simulink model "ALL_JP360_DBW_V6_5_1103"  (R2022a)
settings: Solver=FixedStepAuto  StartTime=0.0  StopTime=inf  FixedStep=0.01  RelTol=1e-3  EnableMultiTasking=on
model workspace (MAT data in the model file):
  g = 9.8
undefined symbols (not defined in the file or in its folder): canChannel, delta_v_p, IPM_Line_C0, IPM_Line_C1, IPM_Line_C2, IPM_Line_C3, M, M_p, MRR_ObjDistX, MRR_ObjDistY, MRR_ObjFusionCamID, MRR_ObjFusionSig, MRR_ObjID, MRR_ObjRelVelX, MRR_ObjRelVelY, MRR_ObjType, MRR_ObjUpdFlg, none, obj_vaild, untracktime, V, videoinput
libraries: canfdmsglib x230, canfdlib x76, slpidlib x24, simulink x18, dspstat3 x14, ctrlSharedLib x1, simulink_extras x1, imaqlib x1, realtime_pacer_lib x1, dspvision x1, visionsinks x1
(part 10 of 55)

== system ALL_JP360_DBW_V6_5_1103/MsgFromCAN/CCAN_ADCU_MsgFromCAN/CCAN_ADCU_ESP_Pressure_0x241 ==
  CCAN_ADCU_ESP_Pressure_0x241FromInData : Inport  OutDataTypeStr=Bus:CAN_FD_MESSAGE_BUS
  Bus Creator : BusCreator  Inputs=11  OutDataTypeStr=Bus:CCAN_ADCU_ESP_Pressure_0x241  NonVirtualBus=on
  CAN FD Unpack : canfdmsglib/CAN FD Unpack  CANdbFile=HiFire_JPT360_CCAN_Matrix_CAN_V1.72_VP_ADCU.dbc  MsgList=(none)  MsgName=ESP_Pressure_0x241  ProtocolMode=CAN FD  MsgIDType=Standard (11-bit identifier)  MsgIdentifier=577  MsgLength=8  SignalInfo={'ABS_ForbidRegen_Active','54','1','BE','unsigned','Standard','0','1','0','0','1';'Checksum_0x241','56','8','BE','unsigned','Standard','0','1','0','0','255';'ESP_Master_Cylinder_Pressure','12','12','BE','unsigned','Standard','0','0.0625','0','0','255.9375';'ESP_Master_Cylinder_Pressure_Status','55','1','BE','unsigned','Standard','0','1','0','0','1';'ESP_MbRegenTargetWhl','32','16','BE','unsigned','Standard','0','1','-30000','-30000','30000';'ESP_MbRegenTargetWhlQualifier','52','2','BE','unsigned','Standard','0','1','0','0','2';'ESP_PresOffsetMasterCylinder','43','5','BE','unsigned','Standard','0','1','-15','-15','15';'ESP_PresOffsetMasterCylinderValid','42','1','BE','unsigned','Standard','0','1','0','0','1';'ESP_TrfCaseModReqdByEsp','40','2','BE','unsigned','Standard','0','1','0','0','3';'ESP_TrfCaseTqLmtdByEsp','16','12','BE','unsigned','Standard','0','1','0','0','4095';'RollingCounter_0x241','48','4','BE','unsigned','Standard','0','1','0','0','15'}  IDPort=off  TimestampPort=off  ErrorPort=off  RemotePort=off  LengthPort=off  StatusPort=off  BRSPort=off  ESIPort=off  DLCPort=off  ApplyMinMax=off
      settings: SourceProductBaseCode=XP,ME,VN  DataFormat=CANdb specified signals
  Data Type Conversion1 : DataTypeConversion  OutDataTypeStr=boolean  SaturateOnIntegerOverflow=off  RndMeth=Floor
  Data Type Conversion10 : DataTypeConversion  OutDataTypeStr=int16  SaturateOnIntegerOverflow=off  RndMeth=Floor
  Data Type Conversion{6..7,9,11} (4 alike) : DataTypeConversion  OutDataTypeStr=int8  SaturateOnIntegerOverflow=off  RndMeth=Floor
  Data Type Conversion2 : DataTypeConversion  OutDataTypeStr=uint8  SaturateOnIntegerOverflow=off  RndMeth=Floor
  Data Type Conversion3 : DataTypeConversion  OutDataTypeStr=single  SaturateOnIntegerOverflow=off  RndMeth=Floor
  Data Type Conversion4 : DataTypeConversion  OutDataTypeStr=boolean  SaturateOnIntegerOverflow=off  RndMeth=Floor
  Data Type Conversion5 : DataTypeConversion  OutDataTypeStr=int16  SaturateOnIntegerOverflow=off  RndMeth=Floor
  Data Type Conversion8 : DataTypeConversion  OutDataTypeStr=boolean  SaturateOnIntegerOverflow=off  RndMeth=Floor
  CCAN_ADCU_ESP_Pressure_0x241FromOutData : Outport  OutDataTypeStr=Bus:CCAN_ADCU_ESP_Pressure_0x241
  wires:
  CAN FD Unpack/1 -> Data Type Conversion1/1
  CAN FD Unpack/2 -> Data Type Conversion2/1
  CAN FD Unpack/3 -> Data Type Conversion3/1
  CAN FD Unpack/4 -> Data Type Conversion4/1
  CAN FD Unpack/5 -> Data Type Conversion5/1
  CAN FD Unpack/6 -> Data Type Conversion6/1
  CAN FD Unpack/7 -> Data Type Conversion7/1
  CAN FD Unpack/8 -> Data Type Conversion8/1
  CAN FD Unpack/9 -> Data Type Conversion9/1
  CAN FD Unpack/10 -> Data Type Conversion10/1
  CAN FD Unpack/11 -> Data Type Conversion11/1
  Data Type Conversion1/1 -> Bus Creator/1  "ABS_ForbidRegen_Active"
  Data Type Conversion2/1 -> Bus Creator/2  "Checksum_0x241"
  Data Type Conversion3/1 -> Bus Creator/3  "ESP_Master_Cylinder_Pressure"
  Data Type Conversion4/1 -> Bus Creator/4  "ESP_Master_Cylinder_Pressure_Status"
  Data Type Conversion5/1 -> Bus Creator/5  "ESP_MbRegenTargetWhl"
  Data Type Conversion6/1 -> Bus Creator/6  "ESP_MbRegenTargetWhlQualifier"
  Data Type Conversion7/1 -> Bus Creator/7  "ESP_PresOffsetMasterCylinder"
  Data Type Conversion8/1 -> Bus Creator/8  "ESP_PresOffsetMasterCylinderValid"
  Data Type Conversion9/1 -> Bus Creator/9  "ESP_TrfCaseModReqdByEsp"
  Data Type Conversion10/1 -> Bus Creator/10  "ESP_TrfCaseTqLmtdByEsp"
  Data Type Conversion11/1 -> Bus Creator/11  "RollingCounter_0x241"
  Bus Creator/1 -> CCAN_ADCU_ESP_Pressure_0x241FromOutData/1  "CCAN_ADCU_ESP_Pressure_0x241FromOutData"
  CCAN_ADCU_ESP_Pressure_0x241FromInData/1 -> CAN FD Unpack/1  "CCAN_ADCU_ESP_Pressure_0x241FromInData"

== system ALL_JP360_DBW_V6_5_1103/MsgFromCAN/CCAN_ADCU_MsgFromCAN/CCAN_ADCU_ESP_RAW_0x212 ==
  CCAN_ADCU_ESP_RAW_0x212FromInData : Inport  OutDataTypeStr=Bus:CAN_FD_MESSAGE_BUS
  Bus Creator : BusCreator  Inputs=10  OutDataTypeStr=Bus:CCAN_ADCU_ESP_RAW_0x212  NonVirtualBus=on
  CAN FD Unpack : canfdmsglib/CAN FD Unpack  CANdbFile=HiFire_JPT360_CCAN_Matrix_CAN_V1.72_VP_ADCU.dbc  MsgList=(none)  MsgName=ESP_RAW_0x212  ProtocolMode=CAN FD  MsgIDType=Standard (11-bit identifier)  MsgIdentifier=530  MsgLength=8  SignalInfo={'Checksum_0x212','56','8','BE','unsigned','Standard','0','1','0','0','255';'ESP_vxwWheelFLValid','55','1','BE','unsigned','Standard','0','1','0','0','1';'ESP_vxwWheelFRValid','54','1','BE','unsigned','Standard','0','1','0','0','1';'ESP_vxwWheelRLValid','53','1','BE','unsigned','Standard','0','1','0','0','1';'ESP_vxwWheelRRValid','52','1','BE','unsigned','Standard','0','1','0','0','1';'ESP_vxwWheelRawFL','12','12','BE','unsigned','Standard','0','0.05625','0','0','230.2875';'ESP_vxwWheelRawFR','16','12','BE','unsigned','Standard','0','0.05625','0','0','230.2875';'ESP_vxwWheelRawRL','36','12','BE','unsigned','Standard','0','0.05625','0','0','230.2875';'ESP_vxwWheelRawRR','40','12','BE','unsigned','Standard','0','0.05625','0','0','230.2875';'RollingCounter_0x212','48','4','BE','unsigned','Standard','0','1','0','0','15'}  IDPort=off  TimestampPort=off  ErrorPort=off  RemotePort=off  LengthPort=off  StatusPort=off  BRSPort=off  ESIPort=off  DLCPort=off  ApplyMinMax=off
      settings: SourceProductBaseCode=XP,ME,VN  DataFormat=CANdb specified signals
  Data Type Conversion1 : DataTypeConversion  OutDataTypeStr=uint8  SaturateOnIntegerOverflow=off  RndMeth=Floor
  Data Type Conversion10 : DataTypeConversion  OutDataTypeStr=int8  SaturateOnIntegerOverflow=off  RndMeth=Floor
  Data Type Conversion{2..5} (4 alike) : DataTypeConversion  OutDataTypeStr=boolean  SaturateOnIntegerOverflow=off  RndMeth=Floor
  Data Type Conversion{6..9} (4 alike) : DataTypeConversion  OutDataTypeStr=single  SaturateOnIntegerOverflow=off  RndMeth=Floor
  CCAN_ADCU_ESP_RAW_0x212FromOutData : Outport  OutDataTypeStr=Bus:CCAN_ADCU_ESP_RAW_0x212
  wires:
  CAN FD Unpack/1 -> Data Type Conversion1/1
  CAN FD Unpack/2 -> Data Type Conversion2/1
  CAN FD Unpack/3 -> Data Type Conversion3/1
  CAN FD Unpack/4 -> Data Type Conversion4/1
  CAN FD Unpack/5 -> Data Type Conversion5/1
  CAN FD Unpack/6 -> Data Type Conversion6/1
  CAN FD Unpack/7 -> Data Type Conversion7/1
  CAN FD Unpack/8 -> Data Type Conversion8/1
  CAN FD Unpack/9 -> Data Type Conversion9/1
  CAN FD Unpack/10 -> Data Type Conversion10/1
  Data Type Conversion1/1 -> Bus Creator/1  "Checksum_0x212"
  Data Type Conversion2/1 -> Bus Creator/2  "ESP_vxwWheelFLValid"
  Data Type Conversion3/1 -> Bus Creator/3  "ESP_vxwWheelFRValid"
  Data Type Conversion4/1 -> Bus Creator/4  "ESP_vxwWheelRLValid"
  Data Type Conversion5/1 -> Bus Creator/5  "ESP_vxwWheelRRValid"
  Data Type Conversion6/1 -> Bus Creator/6  "ESP_vxwWheelRawFL"
  Data Type Conversion7/1 -> Bus Creator/7  "ESP_vxwWheelRawFR"
  Data Type Conversion8/1 -> Bus Creator/8  "ESP_vxwWheelRawRL"
  Data Type Conversion9/1 -> Bus Creator/9  "ESP_vxwWheelRawRR"
  Data Type Conversion10/1 -> Bus Creator/10  "RollingCounter_0x212"
  Bus Creator/1 -> CCAN_ADCU_ESP_RAW_0x212FromOutData/1  "CCAN_ADCU_ESP_RAW_0x212FromOutData"
  CCAN_ADCU_ESP_RAW_0x212FromInData/1 -> CAN FD Unpack/1  "CCAN_ADCU_ESP_RAW_0x212FromInData"

== system ALL_JP360_DBW_V6_5_1103/MsgFromCAN/CCAN_ADCU_MsgFromCAN/CCAN_ADCU_ESP_Status_0x243 ==
  CCAN_ADCU_ESP_Status_0x243FromInData : Inport  OutDataTypeStr=Bus:CAN_FD_MESSAGE_BUS
  Bus Creator : BusCreator  Inputs=38  OutDataTypeStr=Bus:CCAN_ADCU_ESP_Status_0x243  NonVirtualBus=on
  CAN FD Unpack : canfdmsglib/CAN FD Unpack  CANdbFile=HiFire_JPT360_CCAN_Matrix_CAN_V1.72_VP_ADCU.dbc  MsgList=(none)  MsgName=ESP_Status_0x243  ProtocolMode=CAN FD  MsgIDType=Standard (11-bit identifier)  MsgIdentifier=579  MsgLength=8  SignalInfo={'ABS_HAZActive','2','1','BE','unsigned','Standard','0','1','0','0','1';'Checksum_0x243','56','8','BE','unsigned','Standard','0','1','0','0','255';'EBS_EbsFlgFlt','43','1','BE','unsigned','Standard','0','1','0','0','1';'ESP_ATS_Driving_mode_confirm','28','4','BE','unsigned','Standard','0','1','0','0','15';'ESP_ATS_Fault_mode','27','1','BE','unsigned','Standard','0','1','0','0','1';'ESP_ATS_failure_Lamp','24','3','BE','unsigned','Standard','0','1','0','0','7';'ESP_AVHWarningMessage','20','1','BE','unsigned','Standard','0','1','0','0','1';'ESP_AvhActive','21','1','BE','unsigned','Standard','0','1','0','0','1';'ESP_AvhAvabliable','23','1','BE','unsigned','Standard','0','1','0','0','1';'ESP_AvhStandby','22','1','BE','unsigned','Standard','0','1','0','0','1';'ESP_CCSwitchOff','8','1','BE','unsigned','Standard','0','1','0','0','1';'ESP_CdpActive','15','1','BE','unsigned','Standard','0','1','0','0','1';'ESP_CdpAvailable','14','1','BE','unsigned','Standard','0','1','0','0','1';'ESP_Driving_mode_req','36','4','BE','unsigned','Standard','0','1','0','0','15';'ESP_EPBErrorStatus','6','2','BE','unsigned','Standard','0','1','0','0','3';'ESP_EPBStatus','3','3','BE','unsigned','Standard','0','1','0','0','7';'ESP_EPBWarningMessage1','19','1','BE','unsigned','Standard','0','1','0','0','1';'ESP_EPBWarningMessage2','18','1','BE','unsigned','Standard','0','1','0','0','1';'ESP_EPBWarningMessage3','17','1','BE','unsigned','Standard','0','1','0','0','1';'ESP_ESPInfoLamp','44','1','BE','unsigned','Standard','0','1','0','0','1';'ESP_EspCtrlActv','35','1','BE','unsigned','Standard','0','1','0','0','1';'ESP_EspEnableSts','45','1','BE','unsigned','Standard','0','1','0','0','1';'ESP_GearShiftPrevn','46','2','BE','unsigned','Standard','0','1','0','0','3';'ESP_HBBActive_NBS','16','1','BE','unsigned','Standard','0','1','0','0','1';'ESP_HBBstatus','54','2','BE','unsigned','Standard','0','1','0','0','2';'ESP_HBCActive_NBS','53','1','BE','unsigned','Standard','0','1','0','0','1';'ESP_HDCActive','11','2','BE','unsigned','Standard','0','1','0','0','2';'ESP_HDCAvailable','9','1','BE','unsigned','Standard','0','1','0','0','1';'ESP_HHCActive','1','1','BE','unsigned','Standard','0','1','0','0','1';'ESP_HHCAvailable','0','1','BE','unsigned','Standard','0','1','0','0','1';'ESP_LdmBLC_BLRequestController','13','1','BE','unsigned','Standard','0','1','0','0','1';'ESP_SCMSts','41','2','BE','unsigned','Standard','0','1','0','0','3';'ESP_TcsCtrlActv','34','1','BE','unsigned','Standard','0','1','0','0','1';'ESP_TcsFlgFlt','33','1','BE','unsigned','Standard','0','1','0','0','1';'ESP_VAMstatus','10','1','BE','unsigned','Standard','0','1','0','0','1';'ESP_VdcFlgFlt','32','1','BE','unsigned','Standard','0','1','0','0','1';'RollerBenchModeSts','52','1','BE','unsigned','Standard','0','1','0','0','1';'RollingCounter_0x243','48','4','BE','unsigned','Standard','0','1','0','0','15'}  IDPort=off  TimestampPort=off  ErrorPort=off  RemotePort=off  LengthPort=off  StatusPort=off  BRSPort=off  ESIPort=off  DLCPort=off  ApplyMinMax=off
      settings: SourceProductBaseCode=XP,ME,VN  DataFormat=CANdb specified signals
  Data Type Conversion{1,3,5,7..13,17..22,24,26,28..31,33..37} (27 alike) : DataTypeConversion  OutDataTypeStr=boolean  SaturateOnIntegerOverflow=off  RndMeth=Floor
  Data Type Conversion{4,6,14..16,23,25,27,32,38} (10 alike) : DataTypeConversion  OutDataTypeStr=int8  SaturateOnIntegerOverflow=off  RndMeth=Floor
  Data Type Conversion2 : DataTypeConversion  OutDataTypeStr=uint8  SaturateOnIntegerOverflow=off  RndMeth=Floor
  CCAN_ADCU_ESP_Status_0x243FromOutData : Outport  OutDataTypeStr=Bus:CCAN_ADCU_ESP_Status_0x243
  wires:
  CAN FD Unpack/1 -> Data Type Conversion1/1
  CAN FD Unpack/2 -> Data Type Conversion2/1
  CAN FD Unpack/3 -> Data Type Conversion3/1
  CAN FD Unpack/4 -> Data Type Conversion4/1
  CAN FD Unpack/5 -> Data Type Conversion5/1
  CAN FD Unpack/6 -> Data Type Conversion6/1
  CAN FD Unpack/7 -> Data Type Conversion7/1
  CAN FD Unpack/8 -> Data Type Conversion8/1
  CAN FD Unpack/9 -> Data Type Conversion9/1
  CAN FD Unpack/10 -> Data Type Conversion10/1
  CAN FD Unpack/11 -> Data Type Conversion11/1
  CAN FD Unpack/12 -> Data Type Conversion12/1
  CAN FD Unpack/13 -> Data Type Conversion13/1
  CAN FD Unpack/14 -> Data Type Conversion14/1
  CAN FD Unpack/15 -> Data Type Conversion15/1
  CAN FD Unpack/16 -> Data Type Conversion16/1
  CAN FD Unpack/17 -> Data Type Conversion17/1
  CAN FD Unpack/18 -> Data Type Conversion18/1
  CAN FD Unpack/19 -> Data Type Conversion19/1
  CAN FD Unpack/20 -> Data Type Conversion20/1
  CAN FD Unpack/21 -> Data Type Conversion21/1
  CAN FD Unpack/22 -> Data Type Conversion22/1
  CAN FD Unpack/23 -> Data Type Conversion23/1
  CAN FD Unpack/24 -> Data Type Conversion24/1
  CAN FD Unpack/25 -> Data Type Conversion25/1
  CAN FD Unpack/26 -> Data Type Conversion26/1
  CAN FD Unpack/27 -> Data Type Conversion27/1
  CAN FD Unpack/28 -> Data Type Conversion28/1
  CAN FD Unpack/29 -> Data Type Conversion29/1
  CAN FD Unpack/30 -> Data Type Conversion30/1
  CAN FD Unpack/31 -> Data Type Conversion31/1
  CAN FD Unpack/32 -> Data Type Conversion32/1
  CAN FD Unpack/33 -> Data Type Conversion33/1
  CAN FD Unpack/34 -> Data Type Conversion34/1
  CAN FD Unpack/35 -> Data Type Conversion35/1
  CAN FD Unpack/36 -> Data Type Conversion36/1
  CAN FD Unpack/37 -> Data Type Conversion37/1
  CAN FD Unpack/38 -> Data Type Conversion38/1
  Data Type Conversion1/1 -> Bus Creator/1  "ABS_HAZActive"
  Data Type Conversion2/1 -> Bus Creator/2  "Checksum_0x243"
  Data Type Conversion3/1 -> Bus Creator/3  "EBS_EbsFlgFlt"
  Data Type Conversion4/1 -> Bus Creator/4  "ESP_ATS_Driving_mode_confirm"
  Data Type Conversion5/1 -> Bus Creator/5  "ESP_ATS_Fault_mode"
  Data Type Conversion6/1 -> Bus Creator/6  "ESP_ATS_failure_Lamp"
  Data Type Conversion7/1 -> Bus Creator/7  "ESP_AVHWarningMessage"
  Data Type Conversion8/1 -> Bus Creator/8  "ESP_AvhActive"
  Data Type Conversion9/1 -> Bus Creator/9  "ESP_AvhAvabliable"
  Data Type Conversion10/1 -> Bus Creator/10  "ESP_AvhStandby"
  Data Type Conversion11/1 -> Bus Creator/11  "ESP_CCSwitchOff"
  Data Type Conversion12/1 -> Bus Creator/12  "ESP_CdpActive"
  Data Type Conversion13/1 -> Bus Creator/13  "ESP_CdpAvailable"
  Data Type Conversion14/1 -> Bus Creator/14  "ESP_Driving_mode_req"
  Data Type Conversion15/1 -> Bus Creator/15  "ESP_EPBErrorStatus"
  Data Type Conversion16/1 -> Bus Creator/16  "ESP_EPBStatus"
  Data Type Conversion17/1 -> Bus Creator/17  "ESP_EPBWarningMessage1"
  Data Type Conversion18/1 -> Bus Creator/18  "ESP_EPBWarningMessage2"
  Data Type Conversion19/1 -> Bus Creator/19  "ESP_EPBWarningMessage3"
  Data Type Conversion20/1 -> Bus Creator/20  "ESP_ESPInfoLamp"
  Data Type Conversion21/1 -> Bus Creator/21  "ESP_EspCtrlActv"
  Data Type Conversion22/1 -> Bus Creator/22  "ESP_EspEnableSts"
  Data Type Conversion23/1 -> Bus Creator/23  "ESP_GearShiftPrevn"
  Data Type Conversion24/1 -> Bus Creator/24  "ESP_HBBActive_NBS"
  Data Type Conversion25/1 -> Bus Creator/25  "ESP_HBBstatus"
  Data Type Conversion26/1 -> Bus Creator/26  "ESP_HBCActive_NBS"
  Data Type Conversion27/1 -> Bus Creator/27  "ESP_HDCActive"
  Data Type Conversion28/1 -> Bus Creator/28  "ESP_HDCAvailable"
  Data Type Conversion29/1 -> Bus Creator/29  "ESP_HHCActive"
  Data Type Conversion30/1 -> Bus Creator/30  "ESP_HHCAvailable"
  Data Type Conversion31/1 -> Bus Creator/31  "ESP_LdmBLC_BLRequestController"
  Data Type Conversion32/1 -> Bus Creator/32  "ESP_SCMSts"
  Data Type Conversion33/1 -> Bus Creator/33  "ESP_TcsCtrlActv"
  Data Type Conversion34/1 -> Bus Creator/34  "ESP_TcsFlgFlt"
  Data Type Conversion35/1 -> Bus Creator/35  "ESP_VAMstatus"
  Data Type Conversion36/1 -> Bus Creator/36  "ESP_VdcFlgFlt"
  Data Type Conversion37/1 -> Bus Creator/37  "RollerBenchModeSts"
  Data Type Conversion38/1 -> Bus Creator/38  "RollingCounter_0x243"
  Bus Creator/1 -> CCAN_ADCU_ESP_Status_0x243FromOutData/1  "CCAN_ADCU_ESP_Status_0x243FromOutData"
  CCAN_ADCU_ESP_Status_0x243FromInData/1 -> CAN FD Unpack/1  "CCAN_ADCU_ESP_Status_0x243FromInData"

== system ALL_JP360_DBW_V6_5_1103/MsgFromCAN/CCAN_ADCU_MsgFromCAN/CCAN_ADCU_GW_AWD_0x251 ==
  CCAN_ADCU_GW_AWD_0x251FromInData : Inport  OutDataTypeStr=Bus:CAN_FD_MESSAGE_BUS
  Bus Creator : BusCreator  Inputs=22  OutDataTypeStr=Bus:CCAN_ADCU_GW_AWD_0x251  NonVirtualBus=on
  CAN FD Unpack : canfdmsglib/CAN FD Unpack  CANdbFile=HiFire_JPT360_CCAN_Matrix_CAN_V1.72_VP_ADCU.dbc  MsgList=(none)  MsgName=GW_AWD_0x251  ProtocolMode=CAN FD  MsgIDType=Standard (11-bit identifier)  MsgIdentifier=593  MsgLength=8  SignalInfo={'AWD_ATS_Driving_mode_status','44','4','BE','unsigned','Standard','0','1','0','0','7';'AWD_CluCircuitFltSts','62','2','BE','unsigned','Standard','0','1','0','0','3';'AWD_EMODSensorFaultStatus','4','3','BE','unsigned','Standard','0','1','0','0','7';'AWD_EncoderFlt','61','1','BE','unsigned','Standard','0','1','0','0','1';'AWD_ExternalRequestsIgnored','7','1','BE','unsigned','Standard','0','1','0','0','1';'AWD_MotPosition','56','4','BE','unsigned','Standard','0','1','0','0','15';'AWD_OperationModReq','40','3','BE','unsigned','Standard','0','1','0','0','7';'AWD_RPSPosition','1','3','BE','unsigned','Standard','0','1','0','0','7';'AWD_ShiftFlt','49','1','BE','unsigned','Standard','0','1','0','0','1';'AWD_ShiftStuck','48','1','BE','unsigned','Standard','0','1','0','0','1';'AWD_TrfCase2WDLmpReq','38','2','BE','unsigned','Standard','0','1','0','0','3';'AWD_TrfCase4LowShift','20','1','BE','unsigned','Standard','0','1','0','0','1';'AWD_TrfCase4WDAutoLmpReq','34','2','BE','unsigned','Standard','0','1','0','0','3';'AWD_TrfCase4WDLockLmpReq','36','2','BE','unsigned','Standard','0','1','0','0','3';'AWD_TrfCase4WDLowLmpReq','32','2','BE','unsigned','Standard','0','1','0','0','3';'AWD_TrfCaseCoupTFailsafe','55','1','BE','unsigned','Standard','0','1','0','0','1';'AWD_TrfCaseFlgModChg','43','1','BE','unsigned','Standard','0','1','0','0','1';'AWD_TrfCaseFltLmpReq','22','2','BE','unsigned','Standard','0','1','0','0','3';'AWD_TrfCaseSysType','52','3','BE','unsigned','Standard','0','1','0','0','7';'AWD_TrfCaseTqEstimd','24','12','BE','unsigned','Standard','0','1','0','0','3000';'AWD_TrfCaseTqEstimdAvl','21','1','BE','unsigned','Standard','0','1','0','0','1';'AWD_TrfcaseCoupFltSts','50','2','BE','unsigned','Standard','0','1','0','0','3'}  IDPort=off  TimestampPort=off  ErrorPort=off  RemotePort=off  LengthPort=off  StatusPort=off  BRSPort=off  ESIPort=off  DLCPort=off  ApplyMinMax=off
      settings: SourceProductBaseCode=XP,ME,VN  DataFormat=CANdb specified signals
  Data Type Conversion{1..3,6..8,11,13..15,18..19,22} (13 alike) : DataTypeConversion  OutDataTypeStr=int8  SaturateOnIntegerOverflow=off  RndMeth=Floor
  Data Type Conversion{4..5,9..10,12,16..17,21} (8 alike) : DataTypeConversion  OutDataTypeStr=boolean  SaturateOnIntegerOverflow=off  RndMeth=Floor
  Data Type Conversion20 : DataTypeConversion  OutDataTypeStr=int16  SaturateOnIntegerOverflow=off  RndMeth=Floor
  CCAN_ADCU_GW_AWD_0x251FromOutData : Outport  OutDataTypeStr=Bus:CCAN_ADCU_GW_AWD_0x251
  wires:
  CAN FD Unpack/1 -> Data Type Conversion1/1
  CAN FD Unpack/2 -> Data Type Conversion2/1
  CAN FD Unpack/3 -> Data Type Conversion3/1
  CAN FD Unpack/4 -> Data Type Conversion4/1
  CAN FD Unpack/5 -> Data Type Conversion5/1
  CAN FD Unpack/6 -> Data Type Conversion6/1
  CAN FD Unpack/7 -> Data Type Conversion7/1
  CAN FD Unpack/8 -> Data Type Conversion8/1
  CAN FD Unpack/9 -> Data Type Conversion9/1
  CAN FD Unpack/10 -> Data Type Conversion10/1
  CAN FD Unpack/11 -> Data Type Conversion11/1
  CAN FD Unpack/12 -> Data Type Conversion12/1
  CAN FD Unpack/13 -> Data Type Conversion13/1
  CAN FD Unpack/14 -> Data Type Conversion14/1
  CAN FD Unpack/15 -> Data Type Conversion15/1
  CAN FD Unpack/16 -> Data Type Conversion16/1
  CAN FD Unpack/17 -> Data Type Conversion17/1
  CAN FD Unpack/18 -> Data Type Conversion18/1
  CAN FD Unpack/19 -> Data Type Conversion19/1
  CAN FD Unpack/20 -> Data Type Conversion20/1
  CAN FD Unpack/21 -> Data Type Conversion21/1
  CAN FD Unpack/22 -> Data Type Conversion22/1
  Data Type Conversion1/1 -> Bus Creator/1  "AWD_ATS_Driving_mode_status"
  Data Type Conversion2/1 -> Bus Creator/2  "AWD_CluCircuitFltSts"
  Data Type Conversion3/1 -> Bus Creator/3  "AWD_EMODSensorFaultStatus"
  Data Type Conversion4/1 -> Bus Creator/4  "AWD_EncoderFlt"
  Data Type Conversion5/1 -> Bus Creator/5  "AWD_ExternalRequestsIgnored"
  Data Type Conversion6/1 -> Bus Creator/6  "AWD_MotPosition"
  Data Type Conversion7/1 -> Bus Creator/7  "AWD_OperationModReq"
  Data Type Conversion8/1 -> Bus Creator/8  "AWD_RPSPosition"
  Data Type Conversion9/1 -> Bus Creator/9  "AWD_ShiftFlt"
  Data Type Conversion10/1 -> Bus Creator/10  "AWD_ShiftStuck"
  Data Type Conversion11/1 -> Bus Creator/11  "AWD_TrfCase2WDLmpReq"
  Data Type Conversion12/1 -> Bus Creator/12  "AWD_TrfCase4LowShift"
  Data Type Conversion13/1 -> Bus Creator/13  "AWD_TrfCase4WDAutoLmpReq"
  Data Type Conversion14/1 -> Bus Creator/14  "AWD_TrfCase4WDLockLmpReq"
  Data Type Conversion15/1 -> Bus Creator/15  "AWD_TrfCase4WDLowLmpReq"
  Data Type Conversion16/1 -> Bus Creator/16  "AWD_TrfCaseCoupTFailsafe"
  Data Type Conversion17/1 -> Bus Creator/17  "AWD_TrfCaseFlgModChg"
  Data Type Conversion18/1 -> Bus Creator/18  "AWD_TrfCaseFltLmpReq"
  Data Type Conversion19/1 -> Bus Creator/19  "AWD_TrfCaseSysType"
  Data Type Conversion20/1 -> Bus Creator/20  "AWD_TrfCaseTqEstimd"
  Data Type Conversion21/1 -> Bus Creator/21  "AWD_TrfCaseTqEstimdAvl"
  Data Type Conversion22/1 -> Bus Creator/22  "AWD_TrfcaseCoupFltSts"
  Bus Creator/1 -> CCAN_ADCU_GW_AWD_0x251FromOutData/1  "CCAN_ADCU_GW_AWD_0x251FromOutData"
  CCAN_ADCU_GW_AWD_0x251FromInData/1 -> CAN FD Unpack/1  "CCAN_ADCU_GW_AWD_0x251FromInData"

== system ALL_JP360_DBW_V6_5_1103/MsgFromCAN/CCAN_ADCU_MsgFromCAN/CCAN_ADCU_GW_BCM_Door_0x310 ==
  CCAN_ADCU_GW_BCM_Door_0x310FromInData : Inport  OutDataTypeStr=Bus:CAN_FD_MESSAGE_BUS
  Bus Creator : BusCreator  Inputs=26  OutDataTypeStr=Bus:CCAN_ADCU_GW_BCM_Door_0x310  NonVirtualBus=on
  CAN FD Unpack : canfdmsglib/CAN FD Unpack  CANdbFile=HiFire_JPT360_CCAN_Matrix_CAN_V1.72_VP_ADCU.dbc  MsgList=(none)  MsgName=GW_BCM_Door_0x310  ProtocolMode=CAN FD  MsgIDType=Standard (11-bit identifier)  MsgIdentifier=784  MsgLength=8  SignalInfo={'BCM_AntiTheftSts','16','2','BE','unsigned','Standard','0','1','0','0','3';'BCM_ChargePlugSts','34','2','BE','unsigned','Standard','0','1','0','0','3';'BCM_Checksum_0x310','56','8','BE','unsigned','Standard','0','1','0','0','255';'BCM_DoorLockStsFrntLe','14','2','BE','unsigned','Standard','0','1','0','0','3';'BCM_DoorLockStsFrntRi','12','2','BE','unsigned','Standard','0','1','0','0','3';'BCM_DoorLockStsRearLe','10','2','BE','unsigned','Standard','0','1','0','0','3';'BCM_DoorLockStsRearRi','8','2','BE','unsigned','Standard','0','1','0','0','3';'BCM_DoorLockStsTrunk','25','2','BE','unsigned','Standard','0','1','0','0','3';'BCM_DoorStsFrntLe','6','2','BE','unsigned','Standard','0','1','0','0','3';'BCM_DoorStsFrntRi','4','2','BE','unsigned','Standard','0','1','0','0','3';'BCM_DoorStsRearLe','2','2','BE','unsigned','Standard','0','1','0','0','3';'BCM_DoorStsRearRi','0','2','BE','unsigned','Standard','0','1','0','0','3';'BCM_DoorStsTrunk','27','2','BE','unsigned','Standard','0','1','0','0','3';'BCM_EnginehoodSts','38','2','BE','unsigned','Standard','0','1','0','0','3';'BCM_FrontWiperSts','32','2','BE','unsigned','Standard','0','1','0','0','3';'BCM_LoadSensitivity','18','1','BE','unsigned','Standard','0','1','0','0','1';'BCM_LockUnlockFeedback','19','5','BE','unsigned','Standard','0','1','0','0','31';'BCM_MT_NeutralSensorStss','30','2','BE','unsigned','Standard','0','1','0','0','3';'BCM_PLG_DriverSW','41','2','BE','unsigned','Standard','0','1','0','0','3';'BCM_RearWiperSts','46','2','BE','unsigned','Standard','0','1','0','0','3';'BCM_Reverse_gears','52','2','BE','unsigned','Standard','0','1','0','0','3';'BCM_RollingCounter_0x310','48','4','BE','unsigned','Standard','0','1','0','0','15';'BCM_TrunkDoorPreUnlockSts','29','1','BE','unsigned','Standard','0','1','0','0','1';'BCM_TurnIndicatorSts','54','2','BE','unsigned','Standard','0','1','0','0','3';'BCM_WindowsCMD','43','3','BE','unsigned','Standard','0','1','0','0','3';'BCM_oiltankcapSts','36','2','BE','unsigned','Standard','0','1','0','0','3'}  IDPort=off  TimestampPort=off  ErrorPort=off  RemotePort=off  LengthPort=off  StatusPort=off  BRSPort=off  ESIPort=off  DLCPort=off  ApplyMinMax=off
      settings: SourceProductBaseCode=XP,ME,VN  DataFormat=CANdb specified signals
  Data Type Conversion{1..2,4..15,17..22,24..26} (23 alike) : DataTypeConversion  OutDataTypeStr=int8  SaturateOnIntegerOverflow=off  RndMeth=Floor
  Data Type Conversion16 : DataTypeConversion  OutDataTypeStr=boolean  SaturateOnIntegerOverflow=off  RndMeth=Floor
  Data Type Conversion23 : DataTypeConversion  OutDataTypeStr=boolean  SaturateOnIntegerOverflow=off  RndMeth=Floor
  Data Type Conversion3 : DataTypeConversion  OutDataTypeStr=uint8  SaturateOnIntegerOverflow=off  RndMeth=Floor
  CCAN_ADCU_GW_BCM_Door_0x310FromOutData : Outport  OutDataTypeStr=Bus:CCAN_ADCU_GW_BCM_Door_0x310
  wires:
  CAN FD Unpack/1 -> Data Type Conversion1/1
  CAN FD Unpack/2 -> Data Type Conversion2/1
  CAN FD Unpack/3 -> Data Type Conversion3/1
  CAN FD Unpack/4 -> Data Type Conversion4/1
  CAN FD Unpack/5 -> Data Type Conversion5/1
  CAN FD Unpack/6 -> Data Type Conversion6/1
  CAN FD Unpack/7 -> Data Type Conversion7/1
  CAN FD Unpack/8 -> Data Type Conversion8/1
  CAN FD Unpack/9 -> Data Type Conversion9/1
  CAN FD Unpack/10 -> Data Type Conversion10/1
  CAN FD Unpack/11 -> Data Type Conversion11/1
  CAN FD Unpack/12 -> Data Type Conversion12/1
  CAN FD Unpack/13 -> Data Type Conversion13/1
  CAN FD Unpack/14 -> Data Type Conversion14/1
  CAN FD Unpack/15 -> Data Type Conversion15/1
  CAN FD Unpack/16 -> Data Type Conversion16/1
  CAN FD Unpack/17 -> Data Type Conversion17/1
  CAN FD Unpack/18 -> Data Type Conversion18/1
  CAN FD Unpack/19 -> Data Type Conversion19/1
  CAN FD Unpack/20 -> Data Type Conversion20/1
  CAN FD Unpack/21 -> Data Type Conversion21/1
  CAN FD Unpack/22 -> Data Type Conversion22/1
  CAN FD Unpack/23 -> Data Type Conversion23/1
  CAN FD Unpack/24 -> Data Type Conversion24/1
  CAN FD Unpack/25 -> Data Type Conversion25/1
  CAN FD Unpack/26 -> Data Type Conversion26/1
  Data Type Conversion1/1 -> Bus Creator/1  "BCM_AntiTheftSts"
  Data Type Conversion2/1 -> Bus Creator/2  "BCM_ChargePlugSts"
  Data Type Conversion3/1 -> Bus Creator/3  "BCM_Checksum_0x310"
  Data Type Conversion4/1 -> Bus Creator/4  "BCM_DoorLockStsFrntLe"
  Data Type Conversion5/1 -> Bus Creator/5  "BCM_DoorLockStsFrntRi"
  Data Type Conversion6/1 -> Bus Creator/6  "BCM_DoorLockStsRearLe"
  Data Type Conversion7/1 -> Bus Creator/7  "BCM_DoorLockStsRearRi"
  Data Type Conversion8/1 -> Bus Creator/8  "BCM_DoorLockStsTrunk"
  Data Type Conversion9/1 -> Bus Creator/9  "BCM_DoorStsFrntLe"
  Data Type Conversion10/1 -> Bus Creator/10  "BCM_DoorStsFrntRi"
  Data Type Conversion11/1 -> Bus Creator/11  "BCM_DoorStsRearLe"
  Data Type Conversion12/1 -> Bus Creator/12  "BCM_DoorStsRearRi"
  Data Type Conversion13/1 -> Bus Creator/13  "BCM_DoorStsTrunk"
  Data Type Conversion14/1 -> Bus Creator/14  "BCM_EnginehoodSts"
  Data Type Conversion15/1 -> Bus Creator/15  "BCM_FrontWiperSts"
  Data Type Conversion16/1 -> Bus Creator/16  "BCM_LoadSensitivity"
  Data Type Conversion17/1 -> Bus Creator/17  "BCM_LockUnlockFeedback"
  Data Type Conversion18/1 -> Bus Creator/18  "BCM_MT_NeutralSensorStss"
  Data Type Conversion19/1 -> Bus Creator/19  "BCM_PLG_DriverSW"
  Data Type Conversion20/1 -> Bus Creator/20  "BCM_RearWiperSts"
  Data Type Conversion21/1 -> Bus Creator/21  "BCM_Reverse_gears"
  Data Type Conversion22/1 -> Bus Creator/22  "BCM_RollingCounter_0x310"
  Data Type Conversion23/1 -> Bus Creator/23  "BCM_TrunkDoorPreUnlockSts"
  Data Type Conversion24/1 -> Bus Creator/24  "BCM_TurnIndicatorSts"
  Data Type Conversion25/1 -> Bus Creator/25  "BCM_WindowsCMD"
  Data Type Conversion26/1 -> Bus Creator/26  "BCM_oiltankcapSts"
  Bus Creator/1 -> CCAN_ADCU_GW_BCM_Door_0x310FromOutData/1  "CCAN_ADCU_GW_BCM_Door_0x310FromOutData"
  CCAN_ADCU_GW_BCM_Door_0x310FromInData/1 -> CAN FD Unpack/1  "CCAN_ADCU_GW_BCM_Door_0x310FromInData"

== system ALL_JP360_DBW_V6_5_1103/MsgFromCAN/CCAN_ADCU_MsgFromCAN/CCAN_ADCU_GW_Body_0x321 ==
  CCAN_ADCU_GW_Body_0x321FromInData : Inport  OutDataTypeStr=Bus:CAN_FD_MESSAGE_BUS
  Bus Creator : BusCreator  Inputs=20  OutDataTypeStr=Bus:CCAN_ADCU_GW_Body_0x321  NonVirtualBus=on
  CAN FD Unpack : canfdmsglib/CAN FD Unpack  CANdbFile=HiFire_JPT360_CCAN_Matrix_CAN_V1.72_VP_ADCU.dbc  MsgList=(none)  MsgName=GW_Body_0x321  ProtocolMode=CAN FD  MsgIDType=Standard (11-bit identifier)  MsgIdentifier=801  MsgLength=8  SignalInfo={'BCM_AutolampSts','38','2','BE','unsigned','Standard','0','1','0','0','3';'BCM_BrakeFluidSts','36','2','BE','unsigned','Standard','0','1','0','0','3';'BCM_Driving_mode_req','16','4','BE','unsigned','Standard','0','1','0','0','15';'BCM_FrntFogLmpSts','24','2','BE','unsigned','Standard','0','1','0','0','3';'BCM_HighBeamSts','28','2','BE','unsigned','Standard','0','1','0','0','3';'BCM_LowBeamSts','26','2','BE','unsigned','Standard','0','1','0','0','3';'BCM_MT_NeutralSensorSts','42','2','BE','unsigned','Standard','0','1','0','0','3';'BCM_Mechanical_Hand_Brake','4','2','BE','unsigned','Standard','0','1','0','0','3';'BCM_OutsideTemp','8','8','BE','unsigned','Standard','0','0.75','-48','-48','142.5';'BCM_OutsideTempDig','40','2','BE','unsigned','Standard','0','1','0','0','3';'BCM_PosLmpSts','0','2','BE','unsigned','Standard','0','1','0','0','3';'BCM_PowerMode','22','2','BE','unsigned','Standard','0','1','0','0','3';'BCM_PowerModeInvalid','21','1','BE','unsigned','Standard','0','1','0','0','1';'BCM_RearDef_Status','34','2','BE','unsigned','Standard','0','1','0','0','3';'BCM_RearFogLmpSts','30','2','BE','unsigned','Standard','0','1','0','0','3';'BCM_RequestStopStartStatus_AC','44','2','BE','unsigned','Standard','0','1','0','0','3';'BCM_Reverse_gear','6','2','BE','unsigned','Standard','0','1','0','0','3';'BCM_SS_EnableSts','32','2','BE','unsigned','Standard','0','1','0','0','3';'BCM_Start_Switch','46','2','BE','unsigned','Standard','0','1','0','0','3';'TCM_TrailerConnectionSts','20','1','BE','unsigned','Standard','0','1','0','0','1'}  IDPort=off  TimestampPort=off  ErrorPort=off  RemotePort=off  LengthPort=off  StatusPort=off  BRSPort=off  ESIPort=off  DLCPort=off  ApplyMinMax=off
      settings: SourceProductBaseCode=XP,ME,VN  DataFormat=CANdb specified signals
  Data Type Conversion{1..8,10..12,14..19} (17 alike) : DataTypeConversion  OutDataTypeStr=int8  SaturateOnIntegerOverflow=off  RndMeth=Floor
  Data Type Conversion13 : DataTypeConversion  OutDataTypeStr=boolean  SaturateOnIntegerOverflow=off  RndMeth=Floor
  Data Type Conversion20 : DataTypeConversion  OutDataTypeStr=boolean  SaturateOnIntegerOverflow=off  RndMeth=Floor
  Data Type Conversion9 : DataTypeConversion  OutDataTypeStr=single  SaturateOnIntegerOverflow=off  RndMeth=Floor
  CCAN_ADCU_GW_Body_0x321FromOutData : Outport  OutDataTypeStr=Bus:CCAN_ADCU_GW_Body_0x321
  wires:
  CAN FD Unpack/1 -> Data Type Conversion1/1
  CAN FD Unpack/2 -> Data Type Conversion2/1
  CAN FD Unpack/3 -> Data Type Conversion3/1
  CAN FD Unpack/4 -> Data Type Conversion4/1
  CAN FD Unpack/5 -> Data Type Conversion5/1
  CAN FD Unpack/6 -> Data Type Conversion6/1
  CAN FD Unpack/7 -> Data Type Conversion7/1
  CAN FD Unpack/8 -> Data Type Conversion8/1
  CAN FD Unpack/9 -> Data Type Conversion9/1
  CAN FD Unpack/10 -> Data Type Conversion10/1
  CAN FD Unpack/11 -> Data Type Conversion11/1
  CAN FD Unpack/12 -> Data Type Conversion12/1
  CAN FD Unpack/13 -> Data Type Conversion13/1
  CAN FD Unpack/14 -> Data Type Conversion14/1
  CAN FD Unpack/15 -> Data Type Conversion15/1
  CAN FD Unpack/16 -> Data Type Conversion16/1
  CAN FD Unpack/17 -> Data Type Conversion17/1
  CAN FD Unpack/18 -> Data Type Conversion18/1
  CAN FD Unpack/19 -> Data Type Conversion19/1
  CAN FD Unpack/20 -> Data Type Conversion20/1
  Data Type Conversion1/1 -> Bus Creator/1  "BCM_AutolampSts"
  Data Type Conversion2/1 -> Bus Creator/2  "BCM_BrakeFluidSts"
  Data Type Conversion3/1 -> Bus Creator/3  "BCM_Driving_mode_req"
  Data Type Conversion4/1 -> Bus Creator/4  "BCM_FrntFogLmpSts"
  Data Type Conversion5/1 -> Bus Creator/5  "BCM_HighBeamSts"
  Data Type Conversion6/1 -> Bus Creator/6  "BCM_LowBeamSts"
  Data Type Conversion7/1 -> Bus Creator/7  "BCM_MT_NeutralSensorSts"
  Data Type Conversion8/1 -> Bus Creator/8  "BCM_Mechanical_Hand_Brake"
  Data Type Conversion9/1 -> Bus Creator/9  "BCM_OutsideTemp"
  Data Type Conversion10/1 -> Bus Creator/10  "BCM_OutsideTempDig"
  Data Type Conversion11/1 -> Bus Creator/11  "BCM_PosLmpSts"
  Data Type Conversion12/1 -> Bus Creator/12  "BCM_PowerMode"
  Data Type Conversion13/1 -> Bus Creator/13  "BCM_PowerModeInvalid"
  Data Type Conversion14/1 -> Bus Creator/14  "BCM_RearDef_Status"
  Data Type Conversion15/1 -> Bus Creator/15  "BCM_RearFogLmpSts"
  Data Type Conversion16/1 -> Bus Creator/16  "BCM_RequestStopStartStatus_AC"
  Data Type Conversion17/1 -> Bus Creator/17  "BCM_Reverse_gear"
  Data Type Conversion18/1 -> Bus Creator/18  "BCM_SS_EnableSts"
  Data Type Conversion19/1 -> Bus Creator/19  "BCM_Start_Switch"
  Data Type Conversion20/1 -> Bus Creator/20  "TCM_TrailerConnectionSts"
  Bus Creator/1 -> CCAN_ADCU_GW_Body_0x321FromOutData/1  "CCAN_ADCU_GW_Body_0x321FromOutData"
  CCAN_ADCU_GW_Body_0x321FromInData/1 -> CAN FD Unpack/1  "CCAN_ADCU_GW_Body_0x321FromInData"

== system ALL_JP360_DBW_V6_5_1103/MsgFromCAN/CCAN_ADCU_MsgFromCAN/CCAN_ADCU_GW_DMS_0x4A0 ==
  CCAN_ADCU_GW_DMS_0x4A0FromInData : Inport  OutDataTypeStr=Bus:CAN_FD_MESSAGE_BUS
  Bus Creator : BusCreator  Inputs=12  OutDataTypeStr=Bus:CCAN_ADCU_GW_DMS_0x4A0  NonVirtualBus=on
  CAN FD Unpack : canfdmsglib/CAN FD Unpack  CANdbFile=HiFire_JPT360_CCAN_Matrix_CAN_V1.72_VP_ADCU.dbc  MsgList=(none)  MsgName=GW_DMS_0x4A0  ProtocolMode=CAN FD  MsgIDType=Standard (11-bit identifier)  MsgIdentifier=1184  MsgLength=8  SignalInfo={'Checksum_0x4A0','56','8','BE','unsigned','Standard','0','1','0','0','255';'DMS_DriverActionState','24','4','BE','unsigned','Standard','0','1','0','0','7';'DMS_DriverAttentionState','52','3','BE','unsigned','Standard','0','1','0','0','7';'DMS_DriverDrowsinessState','0','3','BE','unsigned','Standard','0','1','0','0','7';'DMS_DriverPitch','8','8','BE','unsigned','Standard','0','1','-90','-90','90';'DMS_DriverWatchRegion','28','4','BE','unsigned','Standard','0','1','0','0','15';'DMS_DriverYaw','16','8','BE','unsigned','Standard','0','1','-90','-90','90';'DMS_IRSensorState','3','2','BE','unsigned','Standard','0','1','0','0','3';'DMS_System_Status','5','3','BE','unsigned','Standard','0','1','0','0','5';'Distraction_Confidence','40','8','BE','unsigned','Standard','0','1','0','0','100';'FatigueWarn_Confidence','32','8','BE','unsigned','Standard','0','1','0','0','100';'RollingCounter_0x4A0','48','4','BE','unsigned','Standard','0','1','0','0','15'}  IDPort=off  TimestampPort=off  ErrorPort=off  RemotePort=off  LengthPort=off  StatusPort=off  BRSPort=off  ESIPort=off  DLCPort=off  ApplyMinMax=off
      settings: SourceProductBaseCode=XP,ME,VN  DataFormat=CANdb specified signals
  Data Type Conversion1 : DataTypeConversion  OutDataTypeStr=uint8  SaturateOnIntegerOverflow=off  RndMeth=Floor
  Data Type Conversion{2..12} (11 alike) : DataTypeConversion  OutDataTypeStr=int8  SaturateOnIntegerOverflow=off  RndMeth=Floor
  CCAN_ADCU_GW_DMS_0x4A0FromOutData : Outport  OutDataTypeStr=Bus:CCAN_ADCU_GW_DMS_0x4A0
  wires:
  CAN FD Unpack/1 -> Data Type Conversion1/1
  CAN FD Unpack/2 -> Data Type Conversion2/1
  CAN FD Unpack/3 -> Data Type Conversion3/1
  CAN FD Unpack/4 -> Data Type Conversion4/1
  CAN FD Unpack/5 -> Data Type Conversion5/1
  CAN FD Unpack/6 -> Data Type Conversion6/1
  CAN FD Unpack/7 -> Data Type Conversion7/1
  CAN FD Unpack/8 -> Data Type Conversion8/1
  CAN FD Unpack/9 -> Data Type Conversion9/1
  CAN FD Unpack/10 -> Data Type Conversion10/1
  CAN FD Unpack/11 -> Data Type Conversion11/1
  CAN FD Unpack/12 -> Data Type Conversion12/1
  Data Type Conversion1/1 -> Bus Creator/1  "Checksum_0x4A0"
  Data Type Conversion2/1 -> Bus Creator/2  "DMS_DriverActionState"
  Data Type Conversion3/1 -> Bus Creator/3  "DMS_DriverAttentionState"
  Data Type Conversion4/1 -> Bus Creator/4  "DMS_DriverDrowsinessState"
  Data Type Conversion5/1 -> Bus Creator/5  "DMS_DriverPitch"
  Data Type Conversion6/1 -> Bus Creator/6  "DMS_DriverWatchRegion"
  Data Type Conversion7/1 -> Bus Creator/7  "DMS_DriverYaw"
  Data Type Conversion8/1 -> Bus Creator/8  "DMS_IRSensorState"
  Data Type Conversion9/1 -> Bus Creator/9  "DMS_System_Status"
  Data Type Conversion10/1 -> Bus Creator/10  "Distraction_Confidence"
  Data Type Conversion11/1 -> Bus Creator/11  "FatigueWarn_Confidence"
  Data Type Conversion12/1 -> Bus Creator/12  "RollingCounter_0x4A0"
  Bus Creator/1 -> CCAN_ADCU_GW_DMS_0x4A0FromOutData/1  "CCAN_ADCU_GW_DMS_0x4A0FromOutData"
  CCAN_ADCU_GW_DMS_0x4A0FromInData/1 -> CAN FD Unpack/1  "CCAN_ADCU_GW_DMS_0x4A0FromInData"

== system ALL_JP360_DBW_V6_5_1103/MsgFromCAN/CCAN_ADCU_MsgFromCAN/CCAN_ADCU_GW_EMS_Engstatus_0x142 ==
  CCAN_ADCU_GW_EMS_Engstatus_0x142FromInData : Inport  OutDataTypeStr=Bus:CAN_FD_MESSAGE_BUS
  Bus Creator : BusCreator  Inputs=8  OutDataTypeStr=Bus:CCAN_ADCU_GW_EMS_Engstatus_0x142  NonVirtualBus=on
  CAN FD Unpack : canfdmsglib/CAN FD Unpack  CANdbFile=HiFire_JPT360_CCAN_Matrix_CAN_V1.72_VP_ADCU.dbc  MsgList=(none)  MsgName=GW_EMS_Engstatus_0x142  ProtocolMode=CAN FD  MsgIDType=Standard (11-bit identifier)  MsgIdentifier=322  MsgLength=8  SignalInfo={'DCM_EMS_Checksum_0x142','56','8','BE','unsigned','Standard','0','1','0','0','255';'DCM_EMS_RollingCounter_0x142','48','4','BE','unsigned','Standard','0','1','0','0','15';'EMS_EngOperationStatus','24','3','BE','unsigned','Standard','0','1','0','0','5';'EMS_EngThrottlePosition','32','8','BE','unsigned','Standard','0','0.392','0','0','99.568';'EMS_SetlEngIdleSpeed','27','13','BE','unsigned','Standard','0','0.5','0','0','4095';'EMS_TargetIdleSpeed','9','15','BE','unsigned','Standard','0','0.5','0','0','16383';'EMS_ThrottlePlatePositionError','8','1','BE','unsigned','Standard','0','1','0','0','1';'EMS_indicatedEngTorqWithoutTCU','52','12','BE','unsigned','Standard','0','0.5','-1000','-1000','1000'}  IDPort=off  TimestampPort=off  ErrorPort=off  RemotePort=off  LengthPort=off  StatusPort=off  BRSPort=off  ESIPort=off  DLCPort=off  ApplyMinMax=off
      settings: SourceProductBaseCode=XP,ME,VN  DataFormat=CANdb specified signals
  Data Type Conversion1 : DataTypeConversion  OutDataTypeStr=uint8  SaturateOnIntegerOverflow=off  RndMeth=Floor
  Data Type Conversion2 : DataTypeConversion  OutDataTypeStr=int8  SaturateOnIntegerOverflow=off  RndMeth=Floor
  Data Type Conversion3 : DataTypeConversion  OutDataTypeStr=int8  SaturateOnIntegerOverflow=off  RndMeth=Floor
  Data Type Conversion{4..6,8} (4 alike) : DataTypeConversion  OutDataTypeStr=single  SaturateOnIntegerOverflow=off  RndMeth=Floor
  Data Type Conversion7 : DataTypeConversion  OutDataTypeStr=boolean  SaturateOnIntegerOverflow=off  RndMeth=Floor
  CCAN_ADCU_GW_EMS_Engstatus_0x142FromOutData : Outport  OutDataTypeStr=Bus:CCAN_ADCU_GW_EMS_Engstatus_0x142
  wires:
  CAN FD Unpack/1 -> Data Type Conversion1/1
  CAN FD Unpack/2 -> Data Type Conversion2/1
  CAN FD Unpack/3 -> Data Type Conversion3/1
  CAN FD Unpack/4 -> Data Type Conversion4/1
  CAN FD Unpack/5 -> Data Type Conversion5/1
  CAN FD Unpack/6 -> Data Type Conversion6/1
  CAN FD Unpack/7 -> Data Type Conversion7/1
  CAN FD Unpack/8 -> Data Type Conversion8/1
  Data Type Conversion1/1 -> Bus Creator/1  "DCM_EMS_Checksum_0x142"
  Data Type Conversion2/1 -> Bus Creator/2  "DCM_EMS_RollingCounter_0x142"
  Data Type Conversion3/1 -> Bus Creator/3  "EMS_EngOperationStatus"
  Data Type Conversion4/1 -> Bus Creator/4  "EMS_EngThrottlePosition"
  Data Type Conversion5/1 -> Bus Creator/5  "EMS_SetlEngIdleSpeed"
  Data Type Conversion6/1 -> Bus Creator/6  "EMS_TargetIdleSpeed"
  Data Type Conversion7/1 -> Bus Creator/7  "EMS_ThrottlePlatePositionError"
  Data Type Conversion8/1 -> Bus Creator/8  "EMS_indicatedEngTorqWithoutTCU"
  Bus Creator/1 -> CCAN_ADCU_GW_EMS_Engstatus_0x142FromOutData/1  "CCAN_ADCU_GW_EMS_Engstatus_0x142FromOutData"
  CCAN_ADCU_GW_EMS_Engstatus_0x142FromInData/1 -> CAN FD Unpack/1  "CCAN_ADCU_GW_EMS_Engstatus_0x142FromInData"

== system ALL_JP360_DBW_V6_5_1103/MsgFromCAN/CCAN_ADCU_MsgFromCAN/CCAN_ADCU_GW_EMS_Sts_0x151 ==
  CCAN_ADCU_GW_EMS_Sts_0x151FromInData : Inport  OutDataTypeStr=Bus:CAN_FD_MESSAGE_BUS
  Bus Creator : BusCreator  Inputs=11  OutDataTypeStr=Bus:CCAN_ADCU_GW_EMS_Sts_0x151  NonVirtualBus=on
  CAN FD Unpack : canfdmsglib/CAN FD Unpack  CANdbFile=HiFire_JPT360_CCAN_Matrix_CAN_V1.72_VP_ADCU.dbc  MsgList=(none)  MsgName=GW_EMS_Sts_0x151  ProtocolMode=CAN FD  MsgIDType=Standard (11-bit identifier)  MsgIdentifier=337  MsgLength=8  SignalInfo={'DCM_EMS_Checksum_0x151','56','8','BE','unsigned','Standard','0','1','0','0','255';'DCM_EMS_RollingCounter_0x151','48','4','BE','unsigned','Standard','0','1','0','0','15';'EMS_ATSDrivingModeStatus','33','2','BE','unsigned','Standard','0','1','0','0','3';'EMS_CatalystWarmUpSts','55','1','BE','unsigned','Standard','0','1','0','0','1';'EMS_CruiseControlStatus','52','2','BE','unsigned','Standard','0','1','0','0','3';'EMS_EngBarometricPressure','16','8','BE','unsigned','Standard','0','1','0','0','254';'EMS_EngOffTime','8','16','BE','unsigned','Standard','0','1','0','0','65534';'EMS_EngReqTCUPreAutoStop','54','1','BE','unsigned','Standard','0','1','0','0','1';'EMS_EngineStopStartStatus','35','3','BE','unsigned','Standard','0','1','0','0','7';'EMS_TargCruiseSpeed','40','9','BE','unsigned','Standard','0','0.5','0','0','255';'EMS_VacuumPressure','38','10','BE','unsigned','Standard','0','0.1','-92.7','-92.7','5'}  IDPort=off  TimestampPort=off  ErrorPort=off  RemotePort=off  LengthPort=off  StatusPort=off  BRSPort=off  ESIPort=off  DLCPort=off  ApplyMinMax=off
      settings: SourceProductBaseCode=XP,ME,VN  DataFormat=CANdb specified signals
  Data Type Conversion1 : DataTypeConversion  OutDataTypeStr=uint8  SaturateOnIntegerOverflow=off  RndMeth=Floor
  Data Type Conversion10 : DataTypeConversion  OutDataTypeStr=single  SaturateOnIntegerOverflow=off  RndMeth=Floor
  Data Type Conversion11 : DataTypeConversion  OutDataTypeStr=single  SaturateOnIntegerOverflow=off  RndMeth=Floor
  Data Type Conversion{2..3,5,9} (4 alike) : DataTypeConversion  OutDataTypeStr=int8  SaturateOnIntegerOverflow=off  RndMeth=Floor
  Data Type Conversion4 : DataTypeConversion  OutDataTypeStr=boolean  SaturateOnIntegerOverflow=off  RndMeth=Floor
  Data Type Conversion6 : DataTypeConversion  OutDataTypeStr=uint8  SaturateOnIntegerOverflow=off  RndMeth=Floor
  Data Type Conversion7 : DataTypeConversion  OutDataTypeStr=uint16  SaturateOnIntegerOverflow=off  RndMeth=Floor
  Data Type Conversion8 : DataTypeConversion  OutDataTypeStr=boolean  SaturateOnIntegerOverflow=off  RndMeth=Floor
  CCAN_ADCU_GW_EMS_Sts_0x151FromOutData : Outport  OutDataTypeStr=Bus:CCAN_ADCU_GW_EMS_Sts_0x151
  wires:
  CAN FD Unpack/1 -> Data Type Conversion1/1
  CAN FD Unpack/2 -> Data Type Conversion2/1
  CAN FD Unpack/3 -> Data Type Conversion3/1
  CAN FD Unpack/4 -> Data Type Conversion4/1
  CAN FD Unpack/5 -> Data Type Conversion5/1
  CAN FD Unpack/6 -> Data Type Conversion6/1
  CAN FD Unpack/7 -> Data Type Conversion7/1
  CAN FD Unpack/8 -> Data Type Conversion8/1
  CAN FD Unpack/9 -> Data Type Conversion9/1
  CAN FD Unpack/10 -> Data Type Conversion10/1
  CAN FD Unpack/11 -> Data Type Conversion11/1
  Data Type Conversion1/1 -> Bus Creator/1  "DCM_EMS_Checksum_0x151"
  Data Type Conversion2/1 -> Bus Creator/2  "DCM_EMS_RollingCounter_0x151"
  Data Type Conversion3/1 -> Bus Creator/3  "EMS_ATSDrivingModeStatus"
  Data Type Conversion4/1 -> Bus Creator/4  "EMS_CatalystWarmUpSts"
  Data Type Conversion5/1 -> Bus Creator/5  "EMS_CruiseControlStatus"
  Data Type Conversion6/1 -> Bus Creator/6  "EMS_EngBarometricPressure"
  Data Type Conversion7/1 -> Bus Creator/7  "EMS_EngOffTime"
  Data Type Conversion8/1 -> Bus Creator/8  "EMS_EngReqTCUPreAutoStop"
  Data Type Conversion9/1 -> Bus Creator/9  "EMS_EngineStopStartStatus"
  Data Type Conversion10/1 -> Bus Creator/10  "EMS_TargCruiseSpeed"
  Data Type Conversion11/1 -> Bus Creator/11  "EMS_VacuumPressure"
  Bus Creator/1 -> CCAN_ADCU_GW_EMS_Sts_0x151FromOutData/1  "CCAN_ADCU_GW_EMS_Sts_0x151FromOutData"
  CCAN_ADCU_GW_EMS_Sts_0x151FromInData/1 -> CAN FD Unpack/1  "CCAN_ADCU_GW_EMS_Sts_0x151FromInData"

== system ALL_JP360_DBW_V6_5_1103/MsgFromCAN/CCAN_ADCU_MsgFromCAN/CCAN_ADCU_GW_EMS_TqWhl_0x111 ==
  CCAN_ADCU_GW_EMS_TqWhl_0x111FromInData : Inport  OutDataTypeStr=Bus:CAN_FD_MESSAGE_BUS
  Bus Creator : BusCreator  Inputs=10  OutDataTypeStr=Bus:CCAN_ADCU_GW_EMS_TqWhl_0x111  NonVirtualBus=on
  CAN FD Unpack : canfdmsglib/CAN FD Unpack  CANdbFile=HiFire_JPT360_CCAN_Matrix_CAN_V1.72_VP_ADCU.dbc  MsgList=(none)  MsgName=GW_EMS_TqWhl_0x111  ProtocolMode=CAN FD  MsgIDType=Standard (11-bit identifier)  MsgIdentifier=273  MsgLength=8  SignalInfo={'Checksum_0x111','56','8','BE','unsigned','Standard','0','1','0','0','255';'EMS_Available','38','1','BE','unsigned','Standard','0','1','0','0','1';'EMS_IndicatedACCMesgError','34','2','BE','unsigned','Standard','0','1','0','0','3';'EMS_IndicatedDriverOverride','39','1','BE','unsigned','Standard','0','1','0','0','1';'EMS_IndicatedDriverReqTorq','52','12','BE','unsigned','Standard','0','0.5','-1000','-1000','1000';'EMS_IndicatedDriverReqTorqWhl','8','16','BE','unsigned','Standard','0','1','-30000','-30000','30000';'EMS_IndicatedEngError','36','1','BE','unsigned','Standard','0','1','0','0','1';'EMS_IndicatedRealEngTorqWhl','24','16','BE','unsigned','Standard','0','1','-30000','-30000','30000';'EMS_Request_Response','37','1','BE','unsigned','Standard','0','1','0','0','1';'RollingCounter_0x111','48','4','BE','unsigned','Standard','0','1','0','0','15'}  IDPort=off  TimestampPort=off  ErrorPort=off  RemotePort=off  LengthPort=off  StatusPort=off  BRSPort=off  ESIPort=off  DLCPort=off  ApplyMinMax=off
      settings: SourceProductBaseCode=XP,ME,VN  DataFormat=CANdb specified signals
  Data Type Conversion1 : DataTypeConversion  OutDataTypeStr=uint8  SaturateOnIntegerOverflow=off  RndMeth=Floor
  Data Type Conversion10 : DataTypeConversion  OutDataTypeStr=int8  SaturateOnIntegerOverflow=off  RndMeth=Floor
  Data Type Conversion{2,4,7,9} (4 alike) : DataTypeConversion  OutDataTypeStr=boolean  SaturateOnIntegerOverflow=off  RndMeth=Floor
  Data Type Conversion3 : DataTypeConversion  OutDataTypeStr=int8  SaturateOnIntegerOverflow=off  RndMeth=Floor
  Data Type Conversion5 : DataTypeConversion  OutDataTypeStr=single  SaturateOnIntegerOverflow=off  RndMeth=Floor
  Data Type Conversion6 : DataTypeConversion  OutDataTypeStr=int16  SaturateOnIntegerOverflow=off  RndMeth=Floor
  Data Type Conversion8 : DataTypeConversion  OutDataTypeStr=int16  SaturateOnIntegerOverflow=off  RndMeth=Floor
  CCAN_ADCU_GW_EMS_TqWhl_0x111FromOutData : Outport  OutDataTypeStr=Bus:CCAN_ADCU_GW_EMS_TqWhl_0x111
  wires:
  CAN FD Unpack/1 -> Data Type Conversion1/1
  CAN FD Unpack/2 -> Data Type Conversion2/1
  CAN FD Unpack/3 -> Data Type Conversion3/1
  CAN FD Unpack/4 -> Data Type Conversion4/1
  CAN FD Unpack/5 -> Data Type Conversion5/1
  CAN FD Unpack/6 -> Data Type Conversion6/1
  CAN FD Unpack/7 -> Data Type Conversion7/1
  CAN FD Unpack/8 -> Data Type Conversion8/1
  CAN FD Unpack/9 -> Data Type Conversion9/1
  CAN FD Unpack/10 -> Data Type Conversion10/1
  Data Type Conversion1/1 -> Bus Creator/1  "Checksum_0x111"
  Data Type Conversion2/1 -> Bus Creator/2  "EMS_Available"
  Data Type Conversion3/1 -> Bus Creator/3  "EMS_IndicatedACCMesgError"
  Data Type Conversion4/1 -> Bus Creator/4  "EMS_IndicatedDriverOverride"
  Data Type Conversion5/1 -> Bus Creator/5  "EMS_IndicatedDriverReqTorq"
  Data Type Conversion6/1 -> Bus Creator/6  "EMS_IndicatedDriverReqTorqWhl"
  Data Type Conversion7/1 -> Bus Creator/7  "EMS_IndicatedEngError"
  Data Type Conversion8/1 -> Bus Creator/8  "EMS_IndicatedRealEngTorqWhl"
  Data Type Conversion9/1 -> Bus Creator/9  "EMS_Request_Response"
  Data Type Conversion10/1 -> Bus Creator/10  "RollingCounter_0x111"
  Bus Creator/1 -> CCAN_ADCU_GW_EMS_TqWhl_0x111FromOutData/1  "CCAN_ADCU_GW_EMS_TqWhl_0x111FromOutData"
  CCAN_ADCU_GW_EMS_TqWhl_0x111FromInData/1 -> CAN FD Unpack/1  "CCAN_ADCU_GW_EMS_TqWhl_0x111FromInData"
